simulink model "Robot_IK_Simulation"  (R2020a)
settings: Solver=VariableStepAuto  StartTime=0.0  StopTime=15  RelTol=1e-3
values from neighbouring files (symbols this model uses):
  orientations = [0     0     0 ... (first row only)    [Robot_Params_and_Waypoints_Data.m]
  Ts = 0.1    [Robot_Params_and_Waypoints_Data.m]
  waypointAccels = zeros(size(waypointVels))    [Robot_Params_and_Waypoints_Data.m]
  waypoints = [-homeConfigHomTr(1:3,4)' + eps ... (first row only)    [Robot_Params_and_Waypoints_Data.m]
  waypointTimes = [0 5 6.5 9.5 11 13 15]    [Robot_Params_and_Waypoints_Data.m]
  waypointVels = 0.1 *[0    0    0 ... (first row only)    [Robot_Params_and_Waypoints_Data.m]
libraries: robotcorelib x5, robotmaniplib x1, trajExampleUtils x1
settings Model: SimulationMode=accelerator  Creator=Mirza  LastModifiedBy=Mirza

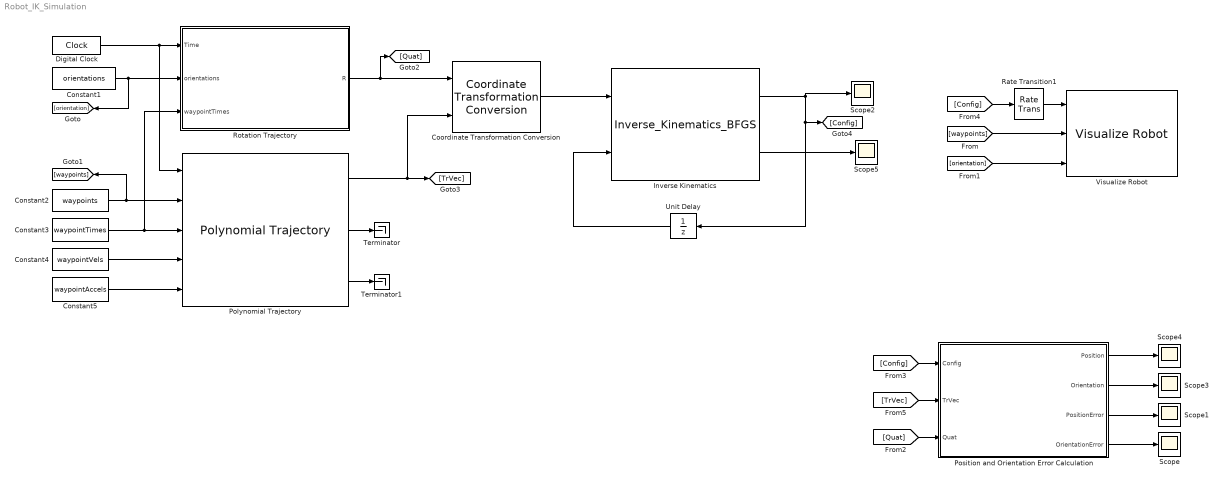
== system Robot_IK_Simulation ==
  Constant1 : Constant  Value=orientations
  Constant2 : Constant  Value=waypoints
  Constant3 : Constant  Value=waypointTimes
  Constant4 : Constant  Value=waypointVels
  Constant5 : Constant  Value=waypointAccels
  Coordinate Transformation Conversion : robotcorelib/Coordinate Transformation Conversion  InputRepresentation=Quaternion  InputEulerSequence=ZYX  ShowTrVecInputPort=on  OutputRepresentation=Homogeneous Transformation  OutputEulerSequence=ZYX  ShowTrVecOutputPort=on  SimulateUsing=Interpreted execution
      settings: SourceProductBaseCode=NV,RO,RR
  Digital Clock : DigitalClock  SampleTime=Ts
  Inverse Kinematics : S-Function  InitFcn=try, set_param(gcb,'FunctionName','Inverse_Kinematics_BFGS'), end  FunctionName=Inverse_Kinematics_BFGS  SFunctionModules=Inverse_Kinematics_BFGS_wrapper  SFunctionDeploymentMode=off  EnableBusSupport=off  mask(S-Function Builder){}
      mask help: Simulink:masks:SFunctionBuilder_MD
      mask init:
      | val = [[.9  0.75 0.75 1 1 .9 .9 1]',[1 1 0.75 0.75 .9 .9 1 .9]'];try , sys = get_param(gcb,'SfunBuilderFcnName');if isempty(sys), sys = get_param(gcb,'FunctionName'); end,catch, sys = get_param(gcb,'FunctionName'); end
      settings: CopyFcn=set_param(gcbh,'LinkStatus','none')  PreSaveFcn=try, set_param(gcb,'FunctionName','Inverse_Kinematics_BFGS'), end  OpenFcn=sfunctionwizard(gcbh)
      mask Display: plot(val(:,1),val(:,2)),disp(sys), port_label('input',1,'Pose'), port_label('input',2,'Init'), port_label('output',1,'Config'), port_label('output',2,'CriterionValue')
  Polynomial Trajectory : robotcorelib/Polynomial Trajectory  WaypointSource=External  Waypoints=[ 0, 2, 1, 5, 0; -1, 3, 1, 4, 4 ]  TimePoints=[ 0, 1, 2, 3, 4 ]  TimeInterval=[ 1, 4 ]  Method=Quintic Polynomial  ParameterSource=External  VelocityBoundaryCondition=zeros( 2, 5 )  AccelerationBoundaryCondition=zeros( 2, 5 )  SimulateUsing=Interpreted execution
      settings: SourceProductBaseCode=NV,RO,RR
  Position and Orientation Error Calculation : Subsystem  Tag=Error Calculation
  Rate Transition1 : RateTransition  OutPortSampleTime=Ts
  Rotation Trajectory : Subsystem
  Scope{,1..5} (6 alike) : Scope
  Terminator : Terminator
  Terminator1 : Terminator
  Unit Delay : UnitDelay  InitialCondition=[0 0 0 0 0 0 0]  SampleTime=-1  HasFrameUpgradeWarning=on
  Visualize Robot : trajExampleUtils/Visualize Robot  rbtName=robotArm  eeName=iiwa_link_ee_kuka  numJoints=numJoints  maxPts=maxWaypoints  plotMode=Coordinate Frames
  wires:
  Polynomial Trajectory/1 -> [TrVec], Coordinate Transformation Conversion/2
  Unit Delay/1 -> Inverse Kinematics/2
  Constant2/1 -> Polynomial Trajectory/2, [waypoints]
  Constant5/1 -> Polynomial Trajectory/5
  Constant4/1 -> Polynomial Trajectory/4
  Digital Clock/1 -> Rotation Trajectory/1(Time), Polynomial Trajectory/1
  Constant3/1 -> Rotation Trajectory/3(waypointTimes), Polynomial Trajectory/3
  Polynomial Trajectory/3 -> Terminator1/1
  Rotation Trajectory/1(R) -> [Quat], Coordinate Transformation Conversion/1
  Constant1/1 -> Rotation Trajectory/2(orientations), [orientation]
  Polynomial Trajectory/2 -> Terminator/1
  Inverse Kinematics/1 -> [Config], Unit Delay/1, Scope2/1
  Rate Transition1/1 -> Visualize Robot/1
  [waypoints] -> Visualize Robot/2
  [orientation] -> Visualize Robot/3
  Coordinate Transformation Conversion/1 -> Inverse Kinematics/1
  Inverse Kinematics/2 -> Scope5/1
  Position and Orientation Error Calculation/1(Position) -> Scope4/1
  Position and Orientation Error Calculation/2(Orientation) -> Scope3/1
  Position and Orientation Error Calculation/4(OrientationError) -> Scope/1
  Position and Orientation Error Calculation/3(PositionError) -> Scope1/1
  [Config] -> Position and Orientation Error Calculation/1(Config)
  [Config] -> Rate Transition1/1
  [TrVec] -> Position and Orientation Error Calculation/2(TrVec)
  [Quat] -> Position and Orientation Error Calculation/3(Quat)

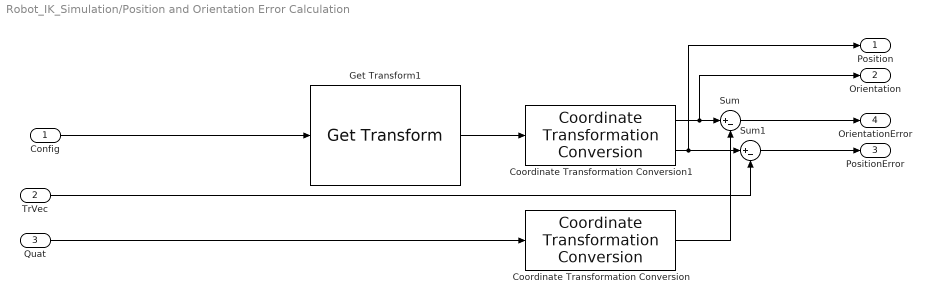
== system Robot_IK_Simulation/Position and Orientation Error Calculation ==
  Config : Inport
  TrVec : Inport  Port=2
  Quat : Inport  Port=3
  Coordinate Transformation Conversion : robotcorelib/Coordinate Transformation Conversion  InputRepresentation=Quaternion  InputEulerSequence=ZYX  ShowTrVecInputPort=on  OutputRepresentation=Euler Angles  OutputEulerSequence=ZYX  ShowTrVecOutputPort=on  SimulateUsing=Interpreted execution
      settings: SourceProductBaseCode=NV,RO,RR
  Coordinate Transformation Conversion1 : robotcorelib/Coordinate Transformation Conversion  InputRepresentation=Homogeneous Transformation  InputEulerSequence=ZYX  ShowTrVecInputPort=on  OutputRepresentation=Euler Angles  OutputEulerSequence=ZYX  ShowTrVecOutputPort=on  SimulateUsing=Interpreted execution
      settings: SourceProductBaseCode=NV,RO,RR
  Get Transform1 : robotmaniplib/Get Transform  RigidBodyTree=robotArm  SourceBody=world  TargetBody=world  SimulateUsing=Interpreted execution
  Sum : Sum  Inputs=|+-
  Sum1 : Sum  Inputs=|+-
  Position : Outport
  Orientation : Outport  Port=2
  PositionError : Outport  Port=3
  OrientationError : Outport  Port=4
  wires:
  Quat/1 -> Coordinate Transformation Conversion/1
  Sum/1 -> OrientationError/1
  Coordinate Transformation Conversion/1 -> Sum/2
  Get Transform1/1 -> Coordinate Transformation Conversion1/1
  Sum1/1 -> PositionError/1
  Coordinate Transformation Conversion1/1 -> Orientation/1, Sum/1
  Coordinate Transformation Conversion1/2 -> Position/1, Sum1/1
  TrVec/1 -> Sum1/2
  Config/1 -> Get Transform1/1

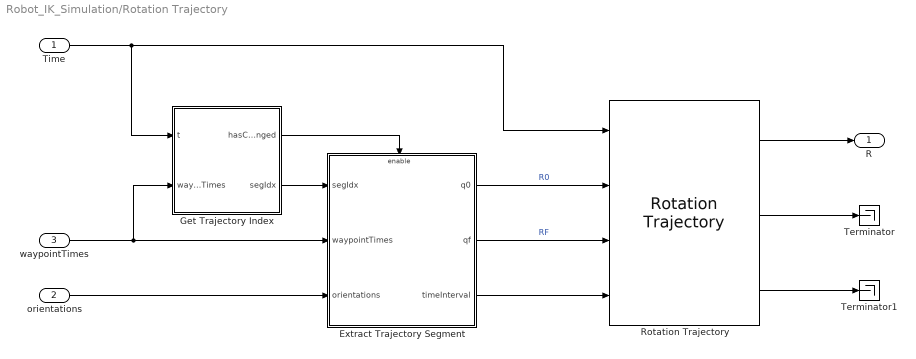
== system Robot_IK_Simulation/Rotation Trajectory ==
  Time : Inport
  orientations : Inport  Port=2
  waypointTimes : Inport  Port=3
  Extract Trajectory Segment : Subsystem
  Get Trajectory Index : MATLAB Function  TreatAsAtomicUnit=on
  Rotation Trajectory : robotcorelib/Rotation Trajectory  WaypointFormat=Quaternion  WaypointSource=External  R0=[ 1, 0, 0, 0 ]'  RF=[ 0, 0, 0, 1 ]'  TimeInterval=[ 0, 4 ]  CustomTimeScaling=off  ParameterSource=Internal  TSTime=0:0.1:1  TimeScaling=[ 0:0.1:1; ones( 1, 11 ); zeros( 1, 11 ) ]  SimulateUsing=Interpreted execution
      settings: SourceProductBaseCode=NV,RO,RR
  Terminator : Terminator
  Terminator1 : Terminator
  R : Outport  VectorParamsAs1DForOutWhenUnconnected=off
  wires:
  Rotation Trajectory/1 -> R/1
  Rotation Trajectory/2 -> Terminator/1
  Rotation Trajectory/3 -> Terminator1/1
  Extract Trajectory Segment/1(q0) -> Rotation Trajectory/2  "R0"
  Extract Trajectory Segment/2(qf) -> Rotation Trajectory/3  "RF"
  Time/1 -> Get Trajectory Index/1(t), Rotation Trajectory/1
  waypointTimes/1 -> Extract Trajectory Segment/2(waypointTimes), Get Trajectory Index/2(waypointTimes)
  Get Trajectory Index/2(segIdx) -> Extract Trajectory Segment/1(segIdx)
  Get Trajectory Index/1(hasChanged) -> Extract Trajectory Segment/Enable
  Extract Trajectory Segment/3(timeInterval) -> Rotation Trajectory/4
  orientations/1 -> Extract Trajectory Segment/3(orientations)

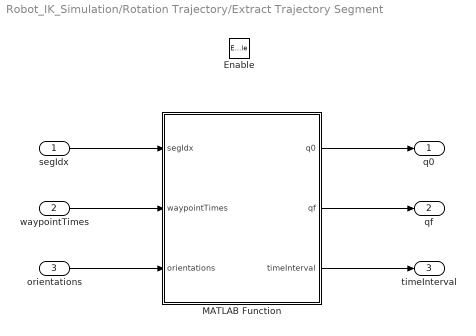
== system Robot_IK_Simulation/Rotation Trajectory/Extract Trajectory Segment ==
  segIdx : Inport
  waypointTimes : Inport  Port=2
  orientations : Inport  Port=3
  Enable : EnablePort  PropagateVarSize=During execution
  MATLAB Function : MATLAB Function  TreatAsAtomicUnit=on
  q0 : Outport  VectorParamsAs1DForOutWhenUnconnected=off
  qf : Outport  Port=2  VectorParamsAs1DForOutWhenUnconnected=off
  timeInterval : Outport  Port=3  VectorParamsAs1DForOutWhenUnconnected=off
  wires:
  segIdx/1 -> MATLAB Function/1(segIdx)
  MATLAB Function/1(q0) -> q0/1
  MATLAB Function/3(timeInterval) -> timeInterval/1
  orientations/1 -> MATLAB Function/3(orientations)
  MATLAB Function/2(qf) -> qf/1
  waypointTimes/1 -> MATLAB Function/2(waypointTimes)

== matlab function Robot_IK_Simulation/Rotation Trajectory/Get Trajectory Index ==
  data: hasChanged output; t input; segIdx output; waypointTimes input size=[1 maxWaypoints]
function [hasChanged,segIdx] = getTrajIdx(t,waypointTimes)

% Initialize previous index
persistent prevIdx
if isempty(prevIdx)
    prevIdx = 0;
end

% Find the trajectory segment index
segIndices = find(t>=waypointTimes);

% Limit the index value to the number of times minus one
% (This addresses the final time case)
segIdx = min(segIndices(end),numel(waypointTimes)-1);

% Determine whether the index has changed from the previous time step
if prevIdx == segIdx
    hasChanged = false;
else
    hasChanged = true;
    prevIdx = segIdx;
end

end

== matlab function Robot_IK_Simulation/Rotation Trajectory/Extract Trajectory Segment/MATLAB Function ==
  data: segIdx input; waypointTimes input size=[1 maxWaypoints]; q0 output size=[1 4]; orientations input size=[3 maxWaypoints]; qf output size=[1 4]; timeInterval output size=[1 2]
function [q0, qf, timeInterval] = createRotationTrajSegment(segIdx,waypointTimes,orientations)

% Extract the time interval, initial, and final quaternions for the segment
timeInterval = waypointTimes(segIdx:segIdx+1);
q0 = eul2quat(orientations(:,segIdx)');
qf = eul2quat(orientations(:,segIdx+1)');

end
